simulink model "rlsdemo"  (Simulink 8.3)
settings: Solver=FixedStepDiscrete  StartTime=0  StopTime=inf  RelTol=1e-3  AbsTol=1e-6
libraries: dspsrcs4 x2, dspsnks4 x1, dspmisc x1, dsparch4 x1, dspadpt3 x1
Description:
  | RLS adaptive noise cancellation
CloseFcn:
  | clear ans;
settings Model: FPTRunName=Active  Creator=The MathWorks Inc.  CovMetricSettings=d  ExtModeTrigMode=oneshot  ExtModeArmWhenConnect=off  ExtModeAutoUpdateStatusClock=off
settings DataIOCC: LimitDataPoints=off  SaveOutput=off  SaveTime=off  SignalLoggingName=sigsOut
settings OptimizationCC: ExpressionDepthLimit=2147483647  InitFltsAndDblsToZero=on  EfficientMapNaN2IntZero=off
settings DebuggingCC: SaveWithParameterizedLinksMsg=none  SignalResolutionControl=TryResolveAllWithWarning  SolverPrmCheckMsg=none  MultiTaskDSMMsg=warning  MultiTaskCondExecSysMsg=none  IntegerOverflowMsg=none  FcnCallInpInsideContextMsg=UseLocalSettings  StrictBusMsg=None
settings HardwareCC: ProdHWDeviceType=Specified  TargetUnknown=on
settings RTWCC: IncludeERTFirstTime=on
settings GRTTargetCC: TargetFcnLib=ansi_tfl_tmw.mat

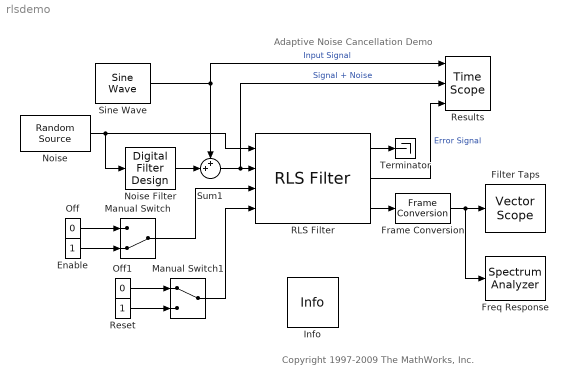
== system rlsdemo ==
  note: Adaptive Noise Cancellation Demo
  note: Copyright 1997-2009 The MathWorks, Inc.
  Enable : Constant  OutDataTypeStr=boolean
  Filter Taps : dspsnks4/Vector Scope  ScopeProperties=off  Domain=User-defined  HorizSpan=1  DisplayProperties=off  AxisGrid=on  Memory=off  FrameNumber=on  AxisLegend=off  AxisZoom=off  OpenScopeAtSimStart=on  OpenScopeImmediately=off  FigPos=[121 62 361 342]  AxisProperties=on  XUnits=Hertz  XRange=[0...Fs/2]  InheritXIncr=on  XIncr=1  XLabel=Samples  XLimit=Auto  XMin=0  XMax=1  XStart=0  YUnits=dB  YLabel=Filter Coefficients  LineProperties=off  LineDisables=on  LineStyles=:  LineMarkers=.  LineColors=[0 0 1]  XAxisParamsVer=6.9
      settings: YMin=-0.2  YMax=0.6
  Frame Conversion : FrameConversion
  Freq Response : SpectrumAnalyzer  ScopeSpecification=DataTag0
  Info : dspmisc/Info  SystemSampleTime=-1
  Manual Switch : ManualSwitch  CurrentSetting=0
  Manual Switch1 : ManualSwitch
  Noise : dspsrcs4/Random Source  SrcType=Gaussian  NormMethod=Ziggurat  CltLength=12  MinVal=0  MaxVal=1  MeanVal=0  VarVal=1  RepMode=Specify seed  rawSeed=[23341]  IsInherit=off  SampMode=Discrete  SampTime=1  SampFrame=1  DataType=Double  OutComplex=Real
  Noise Filter : dsparch4/Digital Filter Design  mwdsp_browser_bugfix_var=off
  Off : Constant  Value=0  OutDataTypeStr=boolean
  Off1 : Constant  Value=0  OutDataTypeStr=boolean
  RLS Filter : dspadpt3/RLS Filter  L=32  lambdaflag=Dialog  lambda=1.0  addnparflag=on  ic=0  delta=0.1  Adapt=on  resetflag=Either edge  weights=on
  Reset : Constant  OutDataTypeStr=boolean
  Results : TimeScope  NumInputPorts=3  DefaultConfigurationName=spbscopes.TimeScopeBlockCfg  ScopeSpecification=DataTag2
  Sine Wave : dspsrcs4/Sine Wave  Amplitude=1  Frequency=0.055  Phase=0  SampleMode=Discrete  OutComplex=Real  CompMethod=Trigonometric fcn  TableSize=Speed  SampleTime=1  SamplesPerFrame=1  ResetState=Restart at time zero  dataType=double  wordLen=16  udDataType=sfix(16)  fracBitsMode=User-defined  numFracBits=14  OutDataTypeStr=double  LastOutDataTypeStr=double
  Sum1 : Sum  Inputs=++|  SaturateOnIntegerOverflow=on  InputSameDT=on  OutDataTypeStr=Inherit: Same as first input
  Terminator : Terminator
  wires:
  Sine Wave/1 -> Results/1, Sum1/1  "Input Signal"
  Noise Filter/1 -> Sum1/2
  Noise/1 -> RLS Filter/1, Noise Filter/1
  Sum1/1 -> RLS Filter/2, Results/2  "Signal + Noise"
  RLS Filter/2 -> Results/3  "Error Signal"
  RLS Filter/1 -> Terminator/1
  Off/1 -> Manual Switch/1
  Enable/1 -> Manual Switch/2
  Off1/1 -> Manual Switch1/1
  Reset/1 -> Manual Switch1/2
  Manual Switch/1 -> RLS Filter/3
  Manual Switch1/1 -> RLS Filter/4
  RLS Filter/3 -> Frame Conversion/1
  Frame Conversion/1 -> Filter Taps/1, Freq Response/1
